simulink model "Simulator_Single_Axis_excitation"  (R2022b)
settings: Solver=ode45  StartTime=0.0  StopTime=simulation_time  RelTol=1e-6  AbsTol=1e-6
values from neighbouring files (symbols this model uses):
  A = [Xu, Xq, -9.81; Mu, Mq, 0; 0, 1, 0]    [Main.m]
  B = [Xd; Md; 0]    [Main.m]
  C = [1, 0, 0; 0, 1, 0; 0, 0, 1; Xu, Xq, 0]    [Main.m]
  D = [0; 0; 0; Xd]    [Main.m]
  sample_time = round(t(end)/length(t),N)    [dis2time_RBS.m]
undefined symbols (not defined in the file or in its folder): BASELINE_T, delay, KD_Q, KD_X_DOT, KI_Q, KI_X_DOT, KP_PITCH, KP_Q, KP_X, KP_X_DOT, N_filter_rate, N_filter_vel, noise, Q_MAX, Q_MIN, VEL_MAX, VEL_MIN
libraries: custom_PIDs_w_reset x2
settings Model: Creator=SalvatoreMeraglia  LastModifiedBy=Lorenzo Miele
settings SolverCC: AlgebraicLoopSolver=TrustRegion
settings DebuggingCC: UnconnectedInputMsg=warning  UnconnectedOutputMsg=warning  UnconnectedLineMsg=warning  SFMachineParentedDataDiag=warning
settings ModelReferenceCC: EnableRefExpFcnMdlSchedulingChecks=on

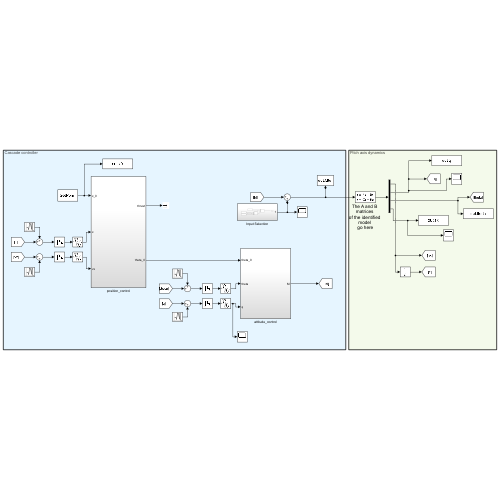
[thumbnail: Simulink's stored preview of the top-level diagram]
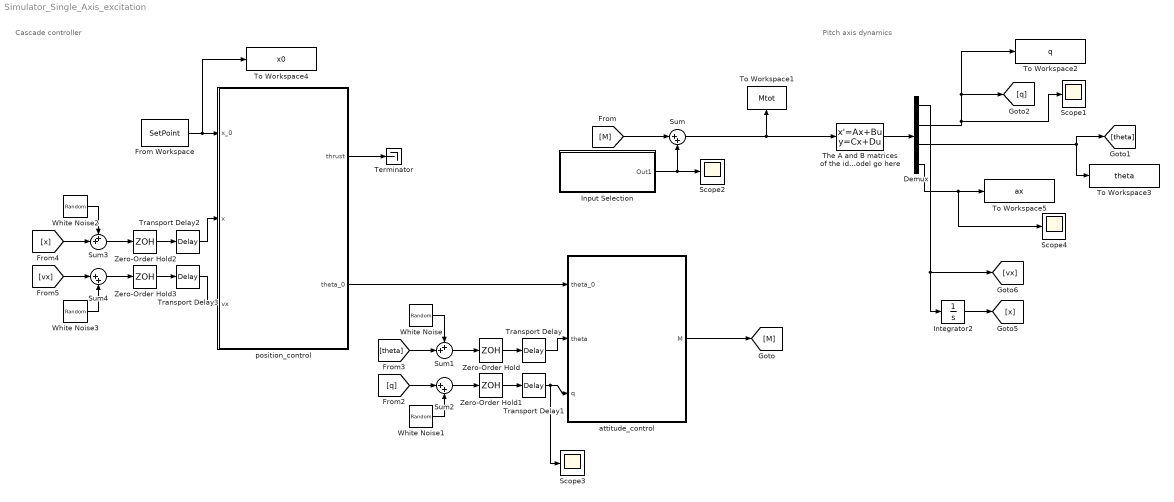
== system Simulator_Single_Axis_excitation ==
  note: Cascade controller
  note: Pitch axis dynamics
  Demux : Demux
  From Workspace : FromWorkspace  VariableName=SetPoint  SampleTime=sample_time  OutputAfterFinalValue=Setting to zero
  Input Selection : Subsystem
  Integrator2 : Integrator
  Scope{1..4} (4 alike) : Scope
  Sum : Sum  Inputs=|++
  Sum1 : Sum  Inputs=++|
  Sum2 : Sum  Inputs=|++
  Sum3 : Sum  Inputs=++|
  Sum4 : Sum  Inputs=|++
  Terminator : Terminator
  The A and B matrices of the identified model go here : StateSpace  A=A  B=B  C=C  D=D  InitialCondition=0
  To Workspace1 : ToWorkspace  VariableName=Mtot  SampleTime=sample_time
  To Workspace2 : ToWorkspace  VariableName=q  SampleTime=sample_time
  To Workspace3 : ToWorkspace  VariableName=theta  SampleTime=sample_time
  To Workspace4 : ToWorkspace  VariableName=x0  SampleTime=sample_time
  To Workspace5 : ToWorkspace  VariableName=ax  SampleTime=sample_time
  Transport Delay : TransportDelay  DelayTime=delay.attitude_filter * sample_time
  Transport Delay1 : TransportDelay  DelayTime=delay.attitude_filter * sample_time
  Transport Delay2 : TransportDelay  DelayTime=delay.position_filter * sample_time
  Transport Delay3 : TransportDelay  DelayTime=delay.position_filter * sample_time
  White Noise : RandomNumber  DisableCoverage=on  Variance=noise.attitude_stand_dev^2  Seed=3  SampleTime=sample_time
  White Noise1 : RandomNumber  DisableCoverage=on  Variance=noise.ang_rate_stand_dev^2  Seed=4  SampleTime=sample_time
  White Noise2 : RandomNumber  DisableCoverage=on  Variance=noise.pos_stand_dev^2  Seed=1  SampleTime=sample_time
  White Noise3 : RandomNumber  DisableCoverage=on  Variance=noise.vel_stand_dev^2  Seed=2  SampleTime=sample_time
  Zero-Order Hold{,1..3} (4 alike) : ZeroOrderHold  SampleTime=sample_time
  attitude_control : Subsystem
  position_control : Subsystem
  wires:
  Transport Delay2/1 -> position_control/2(x)
  Transport Delay3/1 -> position_control/3(vx)
  attitude_control/1(M) -> [M]
  position_control/2(theta_0) -> attitude_control/1(theta_0)
  position_control/1(thrust) -> Terminator/1
  Demux/3 -> To Workspace3/1, [theta]
  [M] -> Sum/1
  Sum/1 -> The A and B matrices of the identified model go here/1, To Workspace1/1
  From Workspace/1 -> To Workspace4/1, position_control/1(x_0)
  Zero-Order Hold1/1 -> Transport Delay1/1
  White Noise2/1 -> Sum3/1
  [theta] -> Sum1/2
  White Noise/1 -> Sum1/1
  Zero-Order Hold/1 -> Transport Delay/1
  [vx] -> Sum4/1
  White Noise3/1 -> Sum4/2
  Sum3/1 -> Zero-Order Hold2/1
  [x] -> Sum3/2
  Zero-Order Hold2/1 -> Transport Delay2/1
  Sum2/1 -> Zero-Order Hold1/1
  [q] -> Sum2/1
  Zero-Order Hold3/1 -> Transport Delay3/1
  Sum4/1 -> Zero-Order Hold3/1
  Sum1/1 -> Zero-Order Hold/1
  White Noise1/1 -> Sum2/2
  Transport Delay1/1 -> Scope3/1, attitude_control/3(q)
  Transport Delay/1 -> attitude_control/2(theta)
  The A and B matrices of the identified model go here/1 -> Demux/1
  Demux/2 -> Scope1/1, To Workspace2/1, [q]
  Demux/1 -> [vx], Integrator2/1
  Integrator2/1 -> [x]
  Demux/4 -> Scope4/1, To Workspace5/1
  Input Selection/1(Out1) -> Scope2/1, Sum/2

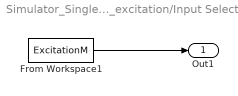
== system Simulator_Single_Axis_excitation/Input Selection ==
  From Workspace1 : FromWorkspace  VariableName=ExcitationM  SampleTime=sample_time  OutputAfterFinalValue=Setting to zero
  Out1 : Outport
  wires:
  From Workspace1/1 -> Out1/1

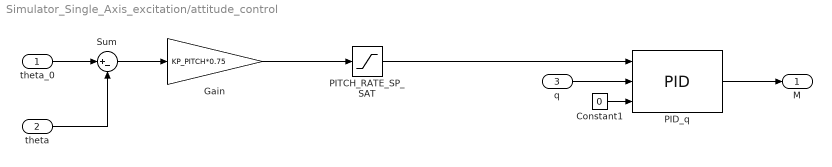
== system Simulator_Single_Axis_excitation/attitude_control ==
  theta_0 : Inport
  theta : Inport  Port=2
  q : Inport  Port=3
  Constant1 : Constant  Value=0  OutDataTypeStr=boolean
  Gain : Gain  Gain=KP_PITCH*0.75
  PID_q : custom_PIDs_w_reset/PID  Kf=KF_Q  Kp=KP_Q  Ki=KI_Q  Kd=KD_Q  N=N_filter_rate  min_u=M_MIN  max_u=M_MAX  ts=sample_time
  PITCH_RATE_SP_SAT : Saturate  UpperLimit=Q_MAX  LowerLimit=Q_MIN
  Sum : Sum  Inputs=|+-
  M : Outport
  wires:
  PID_q/1 -> M/1
  q/1 -> PID_q/2
  PITCH_RATE_SP_SAT/1 -> PID_q/1
  Sum/1 -> Gain/1
  theta_0/1 -> Sum/1
  theta/1 -> Sum/2
  Gain/1 -> PITCH_RATE_SP_SAT/1
  Constant1/1 -> PID_q/3

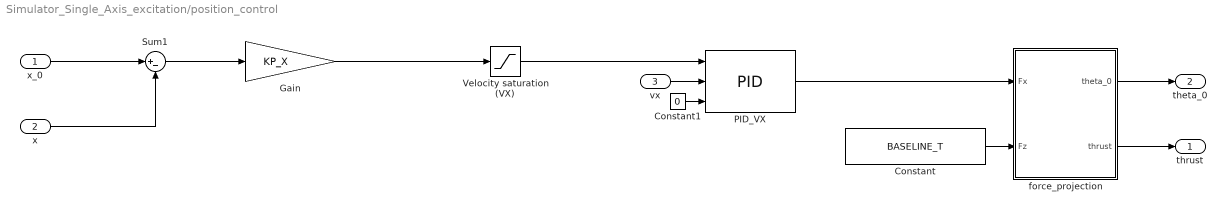
== system Simulator_Single_Axis_excitation/position_control ==
  x_0 : Inport
  x : Inport  Port=2
  vx : Inport  Port=3
  Constant : Constant  Value=BASELINE_T
  Constant1 : Constant  Value=0  OutDataTypeStr=boolean
  Gain : Gain  Gain=KP_X
  PID_VX : custom_PIDs_w_reset/PID  Kf=KF_X_DOT  Kp=KP_X_DOT  Ki=KI_X_DOT  Kd=KD_X_DOT  N=N_filter_vel  min_u=F_X_MIN  max_u=F_X_MAX  ts=sample_time
  Sum1 : Sum  Inputs=|+-
  Velocity saturation (VX) : Saturate  UpperLimit=VEL_MAX  LowerLimit=VEL_MIN
  force_projection : Subsystem
  thrust : Outport
  theta_0 : Outport  Port=2
  wires:
  vx/1 -> PID_VX/2
  Velocity saturation (VX)/1 -> PID_VX/1
  Sum1/1 -> Gain/1
  x_0/1 -> Sum1/1
  x/1 -> Sum1/2
  force_projection/2(thrust) -> thrust/1
  Gain/1 -> Velocity saturation (VX)/1
  Constant1/1 -> PID_VX/3
  Constant/1 -> force_projection/2(Fz)
  PID_VX/1 -> force_projection/1(Fx)
  force_projection/1(theta_0) -> theta_0/1

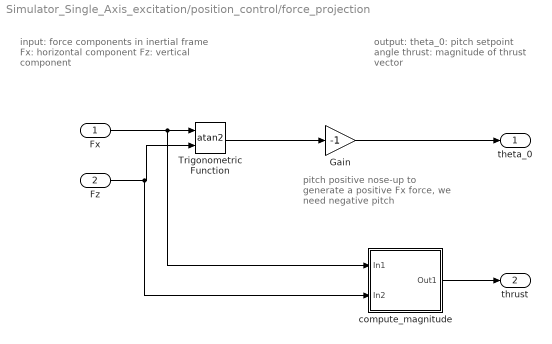
== system Simulator_Single_Axis_excitation/position_control/force_projection ==
  note: pitch positive nose-up
      | to generate a positive Fx force,
      | we need negative pitch
  note: output:
      | theta_0: pitch setpoint angle
      | thrust: magnitude of thrust vector
  note: input: force components in inertial frame
      | Fx: horizontal component
      | Fz: vertical component
  Fx : Inport
  Fz : Inport  Port=2
  Gain : Gain  Gain=-1
  Trigonometric Function : Trigonometry  Operator=atan2
  compute_magnitude : Subsystem
  theta_0 : Outport
  thrust : Outport  Port=2
  wires:
  Fx/1 -> compute_magnitude/1(In1), Trigonometric Function/1
  Fz/1 -> compute_magnitude/2(In2), Trigonometric Function/2
  Trigonometric Function/1 -> Gain/1
  Gain/1 -> theta_0/1
  compute_magnitude/1(Out1) -> thrust/1

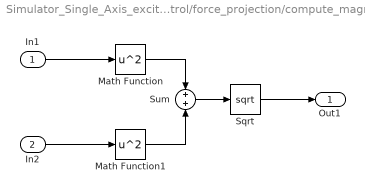
== system Simulator_Single_Axis_excitation/position_control/force_projection/compute_magnitude ==
  In1 : Inport
  In2 : Inport  Port=2
  Math Function : Math  Operator=square  SignedPower=on
  Math Function1 : Math  Operator=square  SignedPower=on
  Sqrt : Sqrt
  Sum : Sum
  Out1 : Outport
  wires:
  Sum/1 -> Sqrt/1
  Sqrt/1 -> Out1/1
  In1/1 -> Math Function/1
  Math Function1/1 -> Sum/2
  Math Function/1 -> Sum/1
  In2/1 -> Math Function1/1
